simulink model "simulation2_eight_old"  (R2017a)
settings: Solver=ode45  StartTime=0.0  StopTime=50  MinStep=0.001  RelTol=1e-3  EnableMultiTasking=on
StopFcn:
  | plotQuadSimResult
values from neighbouring files (symbols this model uses):
  filter = []    [simQuad.m]
  outerController = getOuterController(Ac, 'sedumi')    [main.m]
undefined symbols (not defined in the file or in its folder): quad, sys, us
libraries: simulink x2
settings Model: Creator=cjones  LastModifiedBy=Etienne Clément
settings DataIOCC: LimitDataPoints=on  SaveFormat=Array  SignalLoggingSaveFormat=ModelDataLogs
settings OptimizationCC: ExpressionDepthLimit=2147483647  LifeSpan=inf
settings DebuggingCC: UnderspecifiedInitializationDetection=Classic  MergeDetectMultiDrivingBlocksExec=none  SolverPrmCheckMsg=warning  FcnCallInpInsideContextMsg=warning  StateNameClashWarn=warning  SFUnexpectedBacktrackingDiag=warning  SFNoUnconditionalDefaultTransitionDiag=warning  SFExecutionAtInitializationDiag=none
settings HardwareCC: ProdBitPerPointer=32  ProdBitPerSizeT=32  ProdBitPerPtrDiffT=32  ProdLargestAtomicFloat=None  ProdIntDivRoundTo=Undefined  ProdEndianess=Unspecified  ProdWordSize=32  ProdHWDeviceType=32-bit Generic
settings ModelReferenceCC: PropagateSignalLabelsOutOfModel=off
settings GRTTargetCC: TargetLangStandard=C89/C90 (ANSI)  GeneratePreprocessorConditionals=Disable all  CombineOutputUpdateFcns=off  GRTInterface=on
settings ConfigComp: CovMetricSettings=dw  CovHtmlReporting=on  CovSaveCumulativeToWorkspaceVar=on  CovSaveSingleToWorkspaceVar=on  CovExternalEMLEnable=off

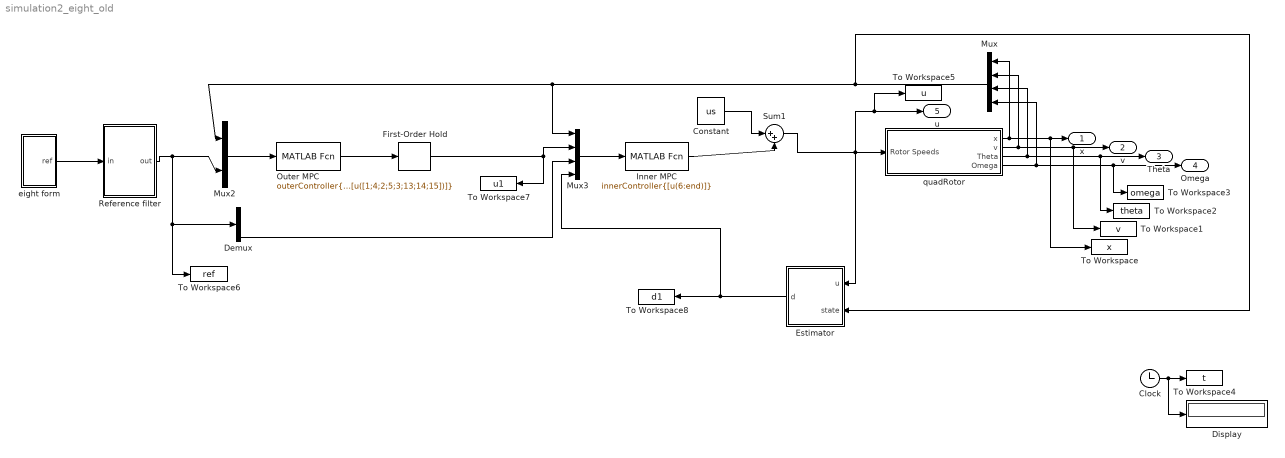
== system simulation2_eight_old ==
  Clock : Clock
  Constant : Constant  Value=us
  Demux : Demux
  Display : Display
  Estimator : Subsystem
  First-Order Hold : simulink/Discrete/First-Order Hold  DisableCoverage=on  Ts=quad.Ts2
      settings: SourceProductName=Simulink  SourceProductBaseCode=SL
  Inner MPC : MATLABFcn  MATLABFcn=innerController{[u(6:end)]}  OutputDimensions=4  OutputSignalType=real  SampleTime=sys.Ts
  Mux : Mux
  Mux2 : Mux  Inputs=[12 4]
  Mux3 : Mux  Inputs=[12 3 1 7]
  Outer MPC : MATLABFcn  MATLABFcn=outerController{[u([1;4;2;5;3;13;14;15])]}  OutputDimensions=3  OutputSignalType=real  SampleTime=quad.Ts2
  Reference filter : Subsystem
  Sum1 : Sum  Inputs=|++
  To Workspace : ToWorkspace  VariableName=x  SampleTime=0.1
  To Workspace1 : ToWorkspace  VariableName=v  SampleTime=0.1
  To Workspace2 : ToWorkspace  VariableName=theta  SampleTime=0.1
  To Workspace3 : ToWorkspace  VariableName=omega  SampleTime=0.1
  To Workspace4 : ToWorkspace  VariableName=t  SampleTime=0.1
  To Workspace5 : ToWorkspace  VariableName=u  SampleTime=0.1
  To Workspace6 : ToWorkspace  VariableName=ref  SampleTime=0.1
  To Workspace7 : ToWorkspace  VariableName=u1  SampleTime=0.1
  To Workspace8 : ToWorkspace  VariableName=d1  SampleTime=0.1
  "eight form " : Subsystem
  quadRotor : Subsystem  mask{dist=on}
      mask prompts: dist "disturbance on/off"
  x : Outport
  v : Outport  Port=2
  Theta : Outport  Port=3
  Omega : Outport  Port=4
  u : Outport  Port=5
  wires:
  quadRotor/1(x) -> x/1, To Workspace/1, Mux/1
  quadRotor/2(v) -> v/1, To Workspace1/1, Mux/2
  quadRotor/4(Omega) -> Omega/1, To Workspace3/1, Mux/4
  quadRotor/3(Theta) -> Mux/3, Theta/1, To Workspace2/1
  Clock/1 -> To Workspace4/1, Display/1
  Mux/1 -> Mux2/1, Mux3/1, Estimator/2(state)
  Demux/4 -> Mux3/3
  Mux3/1 -> Inner MPC/1
  First-Order Hold/1 -> Mux3/2, To Workspace7/1
  Estimator/1(d) -> To Workspace8/1, Mux3/4
  Reference filter/1(out) -> Mux2/2, Demux/1, To Workspace6/1
  Mux2/1 -> Outer MPC/1
  Outer MPC/1 -> First-Order Hold/1
  Constant/1 -> Sum1/1
  Sum1/1 -> To Workspace5/1, u/1, Estimator/1(u), quadRotor/1(Rotor Speeds)
  Inner MPC/1 -> Sum1/2
  "eight form "/1(ref) -> Reference filter/1(in)

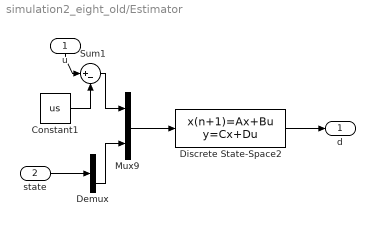
== system simulation2_eight_old/Estimator ==
  u : Inport
  state : Inport  Port=2
  Constant1 : Constant  Value=us
  Demux : Demux  Outputs=[5 7]
  Discrete State-Space2 : DiscreteStateSpace  A=filter.Af  B=filter.Bf  C=[zeros(7,7) eye(7)]  D=zeros(7,11)  SampleTime=sys.Ts
  Mux9 : Mux  Inputs=[4 7]
  Sum1 : Sum  Inputs=|+-
  d : Outport
  wires:
  Mux9/1 -> Discrete State-Space2/1
  Sum1/1 -> Mux9/1
  Constant1/1 -> Sum1/2
  u/1 -> Sum1/1
  state/1 -> Demux/1
  Demux/2 -> Mux9/2
  Discrete State-Space2/1 -> d/1

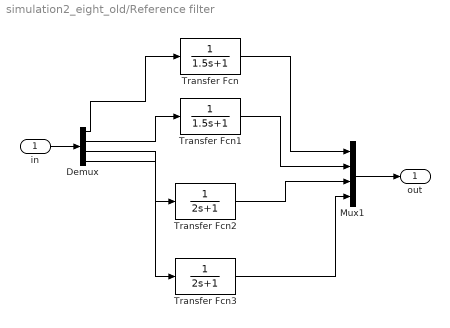
== system simulation2_eight_old/Reference filter ==
  in : Inport
  Demux : Demux
  Mux1 : Mux
  Transfer Fcn : TransferFcn  Denominator=[1.5 1]
  Transfer Fcn1 : TransferFcn  Denominator=[1.5 1]
  Transfer Fcn2 : TransferFcn  Denominator=[2 1]
  Transfer Fcn3 : TransferFcn  Denominator=[2 1]
  out : Outport
  wires:
  Demux/1 -> Transfer Fcn/1
  Demux/2 -> Transfer Fcn1/1
  Demux/3 -> Transfer Fcn2/1
  Demux/4 -> Transfer Fcn3/1
  Mux1/1 -> out/1
  Transfer Fcn/1 -> Mux1/1
  Transfer Fcn1/1 -> Mux1/2
  Transfer Fcn2/1 -> Mux1/3
  Transfer Fcn3/1 -> Mux1/4
  in/1 -> Demux/1

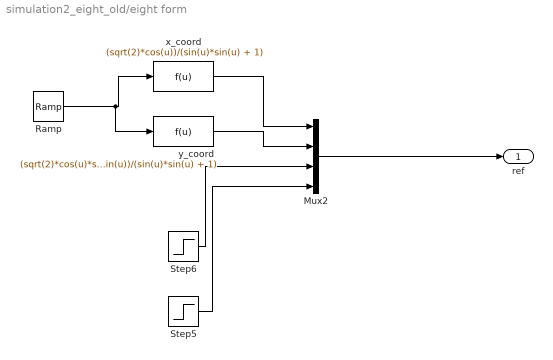
== system simulation2_eight_old/eight form  ==
  Mux2 : Mux
  Ramp : simulink/Sources/Ramp  slope=1  start=0  X0=0
  Step5 : Step  Time=0  After=pi  SampleTime=0
  Step6 : Step  Time=4  After=2  SampleTime=0
  "x_coord " : Fcn  Expr=(sqrt(2)*cos(u))/(sin(u)*sin(u) + 1)
  "y_coord " : Fcn  Expr=(sqrt(2)*cos(u)*sin(u))/(sin(u)*sin(u) + 1)
  ref : Outport
  wires:
  Step6/1 -> Mux2/3
  Step5/1 -> Mux2/4
  Mux2/1 -> ref/1
  Ramp/1 -> "y_coord "/1, "x_coord "/1
  "y_coord "/1 -> Mux2/2
  "x_coord "/1 -> Mux2/1

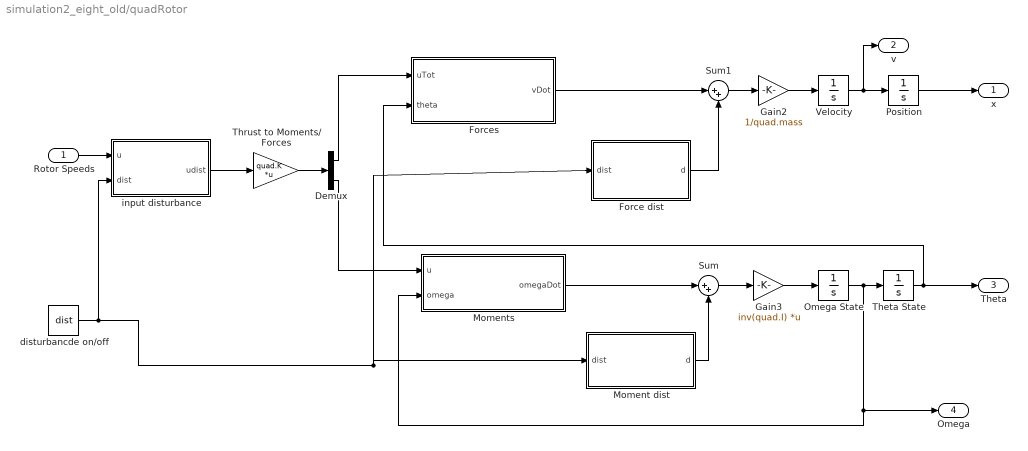
== system simulation2_eight_old/quadRotor ==
  Rotor Speeds : Inport
  Demux : Demux  Outputs=[1 3]
  Force dist : MATLAB Function  TreatAsAtomicUnit=on
  Forces : MATLAB Function  TreatAsAtomicUnit=on
  Gain2 : Gain  Gain=1/quad.mass
  Gain3 : Gain  Gain=inv(quad.I)  Multiplication=Matrix(K*u)
  Moment dist : MATLAB Function  TreatAsAtomicUnit=on  SystemSampleTime=0.05
  Moments : MATLAB Function  TreatAsAtomicUnit=on
  Omega State : Integrator  InitialCondition=[0;0;0]
  Position : Integrator  InitialCondition=[0;0;0]
  Sum : Sum  Inputs=|++
  Sum1 : Sum  Inputs=|++
  Theta State : Integrator  InitialCondition=[0;0;0]
  Thrust to Moments/ Forces : Gain  Gain=quad.K  Multiplication=Matrix(K*u)
  Velocity : Integrator  InitialCondition=[0;0;0]
  disturbancde on/off : Constant  Value=dist
  input disturbance : MATLAB Function  TreatAsAtomicUnit=on
  x : Outport
  v : Outport  Port=2
  Theta : Outport  Port=3
  Omega : Outport  Port=4
  wires:
  Thrust to Moments/ Forces/1 -> Demux/1
  Gain3/1 -> Omega State/1
  Theta State/1 -> Theta/1, Forces/2(theta)
  Demux/1 -> Forces/1(uTot)
  Velocity/1 -> Position/1, v/1
  Rotor Speeds/1 -> input disturbance/1(u)
  Position/1 -> x/1
  Omega State/1 -> Theta State/1, Omega/1, Moments/2(omega)
  Demux/2 -> Moments/1(u)
  Gain2/1 -> Velocity/1
  input disturbance/1(udist) -> Thrust to Moments/ Forces/1
  disturbancde on/off/1 -> input disturbance/2(dist), Force dist/1(dist), Moment dist/1(dist)
  Moment dist/1(d) -> Sum/2
  Moments/1(omegaDot) -> Sum/1
  Sum/1 -> Gain3/1
  Forces/1(vDot) -> Sum1/1
  Sum1/1 -> Gain2/1
  Force dist/1(d) -> Sum1/2

== matlab function simulation2_eight_old/quadRotor/Forces ==
  data: uTot input; vDot output; theta input; quad parameter
function vDot = forces(uTot, theta, quad)
%#codegen

% Rotation from body to interial frame 
roll = theta(1); pitch = theta(2); yaw = theta(3);
R = [1 0 0;0 cos(roll) -sin(roll);0 sin(roll) cos(roll)];
R = R*[cos(pitch) 0 sin(pitch); 0 1 0; -sin(pitch) 0 cos(pitch)];
R = R*[cos(yaw) -sin(yaw) 0; sin(yaw) cos(yaw) 0; 0 0 1];

% Forces
g = 9.81;
vDot = -quad.mass*(g)*[0;0;1] + uTot*R*[0;0;1];

== matlab function simulation2_eight_old/quadRotor/Moments ==
  data: u input; omega input; quad parameter; omegaDot output
function omegaDot = moments(u, omega, quad)
%#codegen
% Rotational derivative
omegaDot = -cross(omega, quad.I*omega) + u ;

== matlab function simulation2_eight_old/quadRotor/input disturbance ==
  data: u input; udist output; dist input
function udist = inputDist(u,dist)
%#codegen
if(dist)
    udist = 1.1*u + 1*[-0.05;0.02;0.03;-0.01];
else
    udist = u;
end

== matlab function simulation2_eight_old/quadRotor/Force dist ==
  data: d output; dist input
function d = forceDist(dist)
%#codegen
if(dist)
    d = -16*[0;0;1]; %gravity error
else
    d = [0;0;0];
end

== matlab function simulation2_eight_old/quadRotor/Moment dist ==
  data: d output; dist input
function d = momentDist(dist)
%#codegen
if(dist)
    d = [1;1;1]  +[0;0;20]*(rand(1)-0.5) + 2*(rand(3,1)-0.5); %disturbance 
else
    d = [0;0;0];
end
